simulink model "rocket_simulation"  (R2024b)
settings: Solver=ode45  StartTime=0.0  StopTime=10.0  RelTol=1e-3
undefined symbols (not defined in the file or in its folder): initialize_rocket_parameters
settings Model: Creator=rishi  LastModifiedBy=rishi

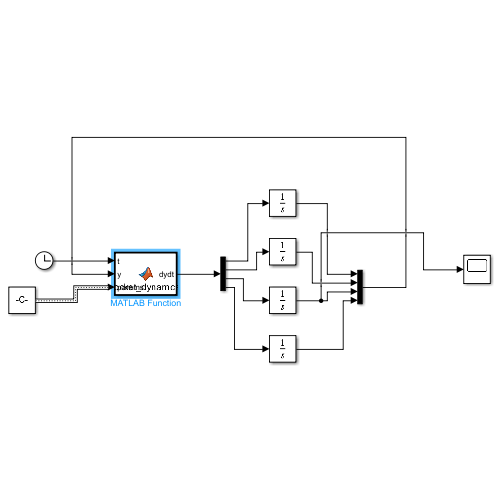
[thumbnail: Simulink's stored preview of the top-level diagram]
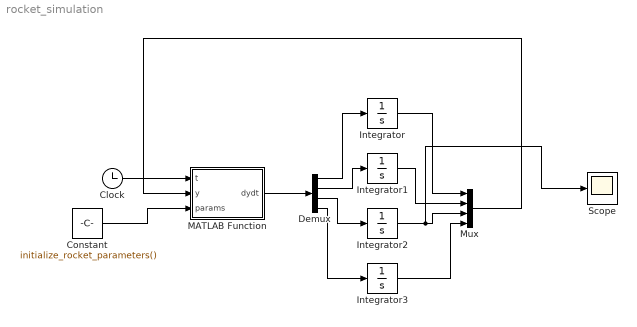
== system rocket_simulation ==
  Clock : Clock
  Constant : Constant  Value=initialize_rocket_parameters()  OutDataTypeStr=Bus: slBus5
  Demux : Demux
  Integrator{,1..3} (4 alike) : Integrator
  MATLAB Function : MATLAB Function  TreatAsAtomicUnit=on
  Mux : Mux
  Scope : Scope
  wires:
  MATLAB Function/1(dydt) -> Demux/1
  Demux/3 -> Integrator2/1
  Demux/4 -> Integrator3/1
  Demux/1 -> Integrator/1
  Demux/2 -> Integrator1/1
  Integrator/1 -> Mux/1
  Integrator1/1 -> Mux/2
  Integrator2/1 -> Scope/1, Mux/3
  Integrator3/1 -> Mux/4
  Mux/1 -> MATLAB Function/2(y)
  Clock/1 -> MATLAB Function/1(t)
  Constant/1 -> MATLAB Function/3(params)

== matlab function rocket_simulation/MATLAB Function ==
  settings: updateMethod=CONTINUOUS
  data: t input; dydt output double size=[4,1]; y input; params input
function dydt = rocket_dynamics(t, y, params)
    dydt = zeros(4,1);
    x = y(1); vx = y(2); alt = y(3); vy = y(4);
    
    % Determine flight phase
    phase = determine_flight_phase(t, alt, vy, params);
    
    % Compute thrust, mass, drag coeff
    [thrust, mass, cd, ref_area] = calculate_forces(t, phase, params);
    
    % Atmosphere & gravity
    [rho, g] = atmosphere_model(alt);
    
    % Wind disturbance (small sinusoidal gust)
    wind = params.wind_amp * sin(2*pi*params.wind_freq*t);
    % in rocket_dynamics, after calculating phase:
    if phase >= 4  % main chute deployed
        effective_wind = params.wind_amp_parachute * sin(2*pi*params.wind_freq*t); % much smaller
    else
        effective_wind = params.wind_amp * sin(2*pi*params.wind_freq*t);
    end

    % Relative velocity
    vrel_x = vx - effective_wind;
    vrel_y = vy;
    vrel = sqrt(vrel_x^2 + vrel_y^2);
    
    % Drag

    Fd = 0.5 * rho * vrel^2 * ref_area * cd;

    if vrel>0
        drag_x = Fd * (vrel_x/vrel);
        drag_y = Fd * (vrel_y/vrel);
    else
        drag_x = 0; drag_y = 0;
    end
    
    % Equations of motion
    dxdt  = vx;
    dvxdt = (thrust*cosd(params.launch_angle) - drag_x) / mass;
    dy_dt  = vy;
    dvydt = (thrust*sind(params.launch_angle) - mass*g - drag_y) / mass;
    
    dydt(1) = dxdt;
    dydt(2) = dvxdt;
    dydt(3) = dy_dt;
    dydt(4) = dvydt;
end

function phase = determine_flight_phase(t, alt, vy, params)
    persistent reached_apogee deployed_drogue deployed_main
    if isempty(reached_apogee),    reached_apogee=false; end
    if isempty(deployed_drogue),    deployed_drogue=false; end
    if isempty(deployed_main),      deployed_main=false; end
    
    if t <= params.burn_time
        phase = 1;                              % powered ascent
    elseif ~reached_apogee && vy<=0
        phase = 2; reached_apogee=true;         % apogee
    elseif reached_apogee && ~deployed_drogue
        phase = 3; deployed_drogue=true;        % drogue deployed at apogee
    elseif reached_apogee && deployed_drogue && ~deployed_main && alt<=params.main_deploy_alt
        phase = 4; deployed_main=true;          % main deployed on descent
    elseif deployed_main
        phase = 5;                              % main-parachute descent
    else
        phase = 2;                              % coasting
    end
end

function [thrust, mass, cd, ref_area] = calculate_forces(t, phase, params)
    switch phase
        case 1  % powered ascent
            thrust = params.max_thrust;
            mass   = params.init_mass - params.mass_flow*t;
            cd     = params.cd_before_main;
            ref_area = params.ref_area_before_main;
        case 2  % coasting to apogee
            thrust = 0;
            mass   = params.dry_mass;
            cd     = params.cd_before_main;
            ref_area = params.ref_area_before_main;
        case 3  % drogue descent
            thrust = 0;
            mass   = params.dry_mass;
            cd     = params.cd_before_main;
            ref_area = params.ref_area_before_main;
        case {4,5}  % main descent (main chute deployed)
            thrust = 0;
            mass   = params.dry_mass;
            cd     = params.cd_after_main;
            ref_area = params.ref_area_after_main;

        otherwise
            thrust = 0;
            mass = 20;
            cd = 0.1;
            ref_area = 0.01;
    end
end

function [rho,g] = atmosphere_model(alt)
    if alt<=11000
        T=288.15-0.0065*alt;
        P=101325*(T/288.15)^5.256;
        rho=P/(287*T);
    else
        rho=0.3639*exp(-0.000157*alt);
    end
    R=6.371e6; g=9.81*(R/(R+alt))^2;
end
